simulink library "ins"  (Simulink 8.1)
settings: Solver=ode1  StartTime=0.0  StopTime=Inf  FixedStep=0.001  RelTol=1e-3
PostLoadFcn:
  | , if any(exist('dsrtsu_mdlpostloadfcn', 'file') == [2, 3, 6]), try dsrtsu_mdlpostloadfcn('Execute', bdroot); catch fprintf('Error in PostLoadFcn (dsrtsu_mdlpostloadfcn) for model "%s":\n %s\n', bdroot, lasterr); end, end,
undefined symbols (not defined in the file or in its folder): AACC_DistCtrlVehSpdError_kph, AACC_VehSpdError_kph, KACC_ACCShortSetTimeGap_s, KACC_DistCtrlIntAddDecel_mps2, MACC_ACCDistIntLookUpDecel_mps2, MACC_ACCDistIntTBLookUpDecel_mps2
libraries: hcu_lib x2
settings Model: DSRTSU_INTERNAL_RTI_VER=450  DSRTSU_INTERNAL_RTI_TYPE=rti1401  Creator=AT015555  LastModifiedBy=AT015555

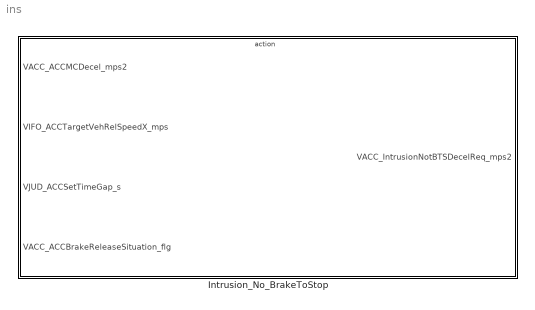
== system ins ==
  Intrusion_No_BrakeToStop : Subsystem  TreatAsAtomicUnit=on

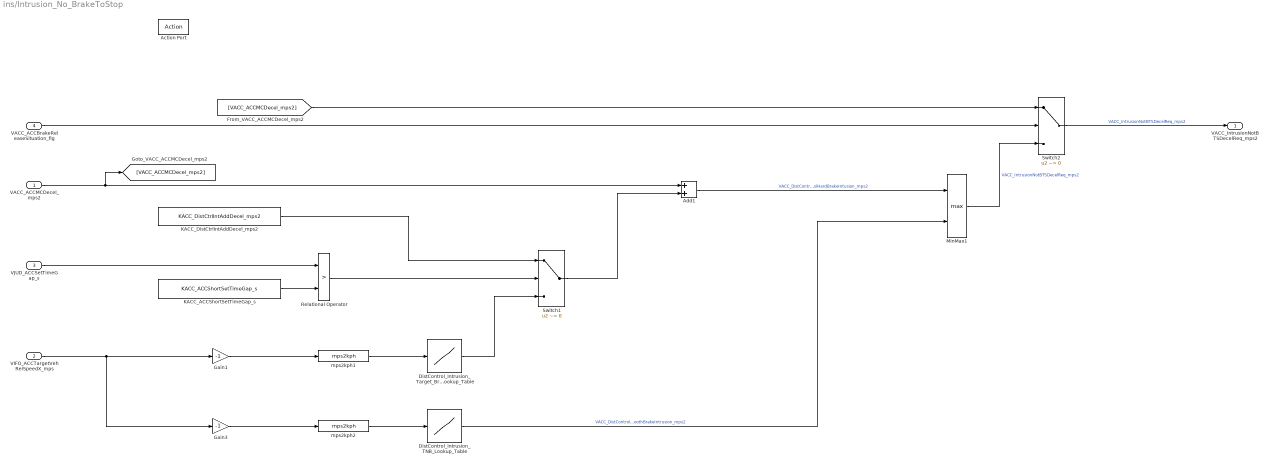
== system ins/Intrusion_No_BrakeToStop ==
  VACC_ACCMCDecel_mps2 : Inport
  VIFO_ACCTargetVehRelSpeedX_mps : Inport  Port=2
  VJUD_ACCSetTimeGap_s : Inport  Port=3
  VACC_ACCBrakeReleaseSituation_flg : Inport  Port=4
  Action Port : ActionPort
  Add1 : Sum
  DistControl_Intrusion_TNB_Lookup_Table : Lookup_n-D  NumberOfTableDimensions=1  BreakpointsForDimension1=AACC_VehSpdError_kph  Table=MACC_ACCDistIntLookUpDecel_mps2  ExtrapMethod=Clip  UseLastTableValue=on  RndMeth=Simplest  InputSameDT=on
  DistControl_Intrusion_Target_Braking_Lookup_Table : Lookup_n-D  NumberOfTableDimensions=1  BreakpointsForDimension1=AACC_DistCtrlVehSpdError_kph  Table=MACC_ACCDistIntTBLookUpDecel_mps2  ExtrapMethod=Clip  UseLastTableValue=on  RndMeth=Simplest  InputSameDT=on
  Gain1 : Gain  Gain=-1
  Gain3 : Gain  Gain=-1
  KACC_ACCShortSetTimeGap_s : Constant  Value=KACC_ACCShortSetTimeGap_s
  KACC_DistCtrlIntAddDecel_mps2 : Constant  Value=KACC_DistCtrlIntAddDecel_mps2
  MinMax1 : MinMax  Function=max  Inputs=2
  Relational Operator : RelationalOperator  Operator=>  OutDataTypeStr=boolean
  Switch1 : Switch  Criteria=u2 ~= 0
  Switch2 : Switch  Criteria=u2 ~= 0
  mps2kph1 : hcu_lib/mps2kph
  mps2kph2 : hcu_lib/mps2kph
  VACC_IntrusionNotBTSDecelReq_mps2 : Outport
  wires:
  Switch2/1 -> VACC_IntrusionNotBTSDecelReq_mps2/1  "VACC_IntrusionNotBTSDecelReq_mps2"
  Gain1/1 -> mps2kph1/1
  mps2kph1/1 -> DistControl_Intrusion_Target_Braking_Lookup_Table/1
  mps2kph2/1 -> DistControl_Intrusion_TNB_Lookup_Table/1
  Gain3/1 -> mps2kph2/1
  VIFO_ACCTargetVehRelSpeedX_mps/1 -> Gain1/1, Gain3/1
  Add1/1 -> MinMax1/1  "VACC_DistControlHardBrakeIntusion_mps2"
  DistControl_Intrusion_TNB_Lookup_Table/1 -> MinMax1/2  "VACC_DistControlTargetSmoothBrakeIntrusion_mps2"
  KACC_DistCtrlIntAddDecel_mps2/1 -> Switch1/1
  Relational Operator/1 -> Switch1/2
  VJUD_ACCSetTimeGap_s/1 -> Relational Operator/1
  KACC_ACCShortSetTimeGap_s/1 -> Relational Operator/2
  Switch1/1 -> Add1/2
  DistControl_Intrusion_Target_Braking_Lookup_Table/1 -> Switch1/3
  VACC_ACCMCDecel_mps2/1 -> [VACC_ACCMCDecel_mps2], Add1/1
  VACC_ACCBrakeReleaseSituation_flg/1 -> Switch2/2
  [VACC_ACCMCDecel_mps2] -> Switch2/1
  MinMax1/1 -> Switch2/3  "VACC_IntrusionNotBTSDecelReq_mps2"
